simulink model "eVTOL_PX4_2023b"  (R2024b)
settings: Solver=ode4  StartTime=0  StopTime=inf  FixedStep=0.01  RelTol=1e-3
values from neighbouring files (symbols this model uses):
  aDl =     [initdata.mat]
  aDr =     [initdata.mat]
  aDyn =     [initdata.mat]
  Airport = init_airport('PHNL')    [initdata_HIL_eVTOL.m]
  aLat =     [initdata.mat]
  aLon =     [initdata.mat]
  D = Prop.D    [EOM_dt_MC.m]    (also in EOM_get_alf_dt_de_prop_evtol.m = CD * QS)
  dt0 = X(2)    [EOM_get_alf_dt_de_prop_evtol.m]    (also in initdata.mat = 0.258252593971; initdata_HIL_eVTOL.m = EOM_dt_MC)
  EAS0 = TAS0 / EAS2TAS    [initdata_HIL_eVTOL.m]
  FCS = init_FCS    [initdata_HIL_eVTOL.m]
  General = init_layoutdata    [EOM_dt_MC.m]    (also in build_optimized_CA.m; initdata.mat = ; initdata_HIL_eVTOL.m)
  h0 = Con(1)    [EOM_get_alf_dt_de_prop_evtol.m]    (also in initdata.mat = 450; initdata_HIL_eVTOL.m = 50)
  mass = Con(3)    [EOM_get_alf_dt_de_prop_evtol.m]    (also in initdata.mat = 2255.54; initdata_HIL_eVTOL.m = 7)
  Motor = init_motor_evtol    [EOM_dt_MC.m]    (also in initdata.mat = []; initdata_HIL_eVTOL.m)
  Prop = init_propeller_evtol_new    [EOM_dt_MC.m]    (also in initdata_HIL_eVTOL.m)
  R2D = 180/pi    (= 57.2957795131)    [EOM_get_alf_dt_de_prop_evtol.m]    (also in init_FCS.m; init_aerodata_evtol.m; init_airport.m; initdata.mat)
  SAMPLE_TIME = 0.01    [initdata_HIL_eVTOL.m]
  theta0 = -0.0510981441662    [initdata.mat]
undefined symbols (not defined in the file or in its folder): A1, aDa, aDe, aero, asbhl20env, B1, C1, de0, Earth, Environment, INIT_Data, InitData, Kd, Kp, magnitude, Newton, pProp, Raphson, Tc, WGS84
libraries: simulink_extras x63, vrlib x48, sharedtransform x28, simulink x22, slpidlib x20, sharedutil x20, matrix_library x18, aerolibwindfilters x12, aerolibobsolete x8, aerolibasang x8, aerolibatmos2 x6, aerolibfltsims x6
(part 11 of 17)

== system eVTOL_PX4_2023b/FCS/FW/TECS/TECS PX4 & AP201/throttlec_AP201 ==
  LonMod : Inport
  SPE_RATE_C : Inport  Port=2
  SKE_RATE_C : Inport  Port=3
  SPE_RATE : Inport  Port=4
  SKE_RATE : Inport  Port=5
  Add2 : Sum  Inputs=++|
  Add6 : Sum  Inputs=++|
  Add7 : Sum  Inputs=++|
  Add9 : Sum  Inputs=+-|
  Detect Change : simulink/Logic and Bit Operations/Detect Change  vinit=0  OutDataTypeStr=boolean
  Divide2 : Product  Inputs=*/
  Integrator1 : Integrator  ExternalReset=either  LimitOutput=on  UpperSaturationLimit=0.5  LowerSaturationLimit=-0.5  ZeroCross=off
  KTI : Gain  Gain=0.8
  KTP : Gain  Gain=0.4
  PX4 1st order filter (time depended)1 : CustomLib/PX4 1st order filter (time depended)  Commented=on  Ts=0.2
  Rate Limiter Dynamic1 : simulink/Discontinuities/Rate Limiter Dynamic
  Saturation Dynamic : simulink/Discontinuities/Saturation Dynamic  OutMin=[]  OutMax=[]  OutDataTypeStr=Inherit: Same as second input  OutDataType=fixdt(1, 16)  OutScaling=2^-10  DoSatur=off
  Saturation3 : Saturate  UpperLimit=1  LowerLimit=-1
  dE_dot scp : Scope
  dt scp{2..5} (4 alike) : Scope
  dt_slew : Constant  Value=0.8
  dti scp1 : Scope  NumInputPorts=2
  g12 : Gain  Gain=9.8
  g13 : Gain  Gain=-1
  dt : Outport  VectorParamsAs1DForOutWhenUnconnected=off
  wires:
  Add2/1 -> Rate Limiter Dynamic1/2  "dt"
  Saturation Dynamic/1 -> dt scp4/1, Add9/1  "STE_rate_c"
  Rate Limiter Dynamic1/1 -> Saturation3/1
  [STE_rate_min] -> Saturation Dynamic/3
  Add7/1 -> dt scp5/1, Saturation Dynamic/2  "STE_rate_c"
  Divide2/1 -> dE_dot scp/1, KTI/1, KTP/1  "dE_dot"
  g12/1 -> Divide2/2
  SPE_RATE/1 -> Add6/1
  Add9/1 -> Divide2/1  "STE_rate_err"
  [V] -> g12/1
  KTI/1 -> Integrator1/1
  SKE_RATE/1 -> Add6/2
  KTP/1 -> Add2/2, dti scp1/2
  Add6/1 -> dt scp3/1, Add9/2  "STE_rate"
  SKE_RATE_C/1 -> Add7/2
  SPE_RATE_C/1 -> Add7/1
  [STE_rate_max] -> Saturation Dynamic/1
  Integrator1/1 -> Add2/1, dti scp1/1
  dt_slew/1 -> Rate Limiter Dynamic1/1, g13/1
  g13/1 -> Rate Limiter Dynamic1/3
  Saturation3/1 -> dt/1, dt scp2/1
  LonMod/1 -> Detect Change/1
  Detect Change/1 -> Integrator1/2

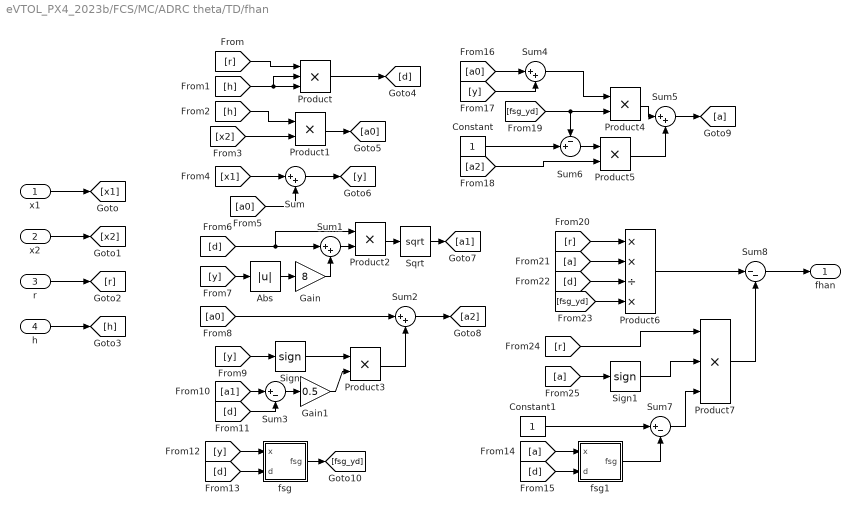
== system eVTOL_PX4_2023b/FCS/MC/ADRC theta/TD/fhan ==
  x1 : Inport
  x2 : Inport  Port=2
  r : Inport  Port=3
  h : Inport  Port=4
  Abs : Abs  SaturateOnIntegerOverflow=off
  Constant : Constant
  Constant1 : Constant
  Gain : Gain  Gain=8
  Gain1 : Gain  Gain=0.5
  Product : Product  Inputs=3
  Product{1..5} (5 alike) : Product
  Product6 : Product  Inputs=**/*
  Product7 : Product  Inputs=***
  Sign : Signum
  Sign1 : Signum
  Sqrt : Sqrt
  Sum{,1..2,4..5} (5 alike) : Sum  Inputs=|++
  Sum3 : Sum  Inputs=|+-
  Sum6 : Sum  Inputs=-+|
  Sum7 : Sum  Inputs=|+-
  Sum8 : Sum  Inputs=|--
  fsg : Subsystem
  fsg1 : Subsystem
  fhan : Outport
  wires:
  Product/1 -> [d]
  x1/1 -> [x1]
  x2/1 -> [x2]
  r/1 -> [r]
  h/1 -> [h]
  [r] -> Product/1
  [h] -> Product/3, Product/2
  [h] -> Product1/1
  [x2] -> Product1/2
  Product1/1 -> [a0]
  [x1] -> Sum/1
  [a0] -> Sum/2
  Sum/1 -> [y]
  [d] -> Sum1/1, Product2/1
  [y] -> Abs/1
  Abs/1 -> Gain/1
  Gain/1 -> Sum1/2
  Sum1/1 -> Product2/2
  Product2/1 -> Sqrt/1
  [a0] -> Sum2/1
  [y] -> Sign/1
  Sign/1 -> Product3/1
  [a1] -> Sum3/1
  [d] -> Sum3/2
  Sum3/1 -> Gain1/1
  Gain1/1 -> Product3/2
  Product3/1 -> Sum2/2
  Sum2/1 -> [a2]
  [y] -> fsg/1(x)
  [d] -> fsg/2(d)
  [d] -> fsg1/2(d)
  [a] -> fsg1/1(x)
  [a0] -> Sum4/1
  [y] -> Sum4/2
  Sum4/1 -> Product4/1
  Product4/1 -> Sum5/1
  [a2] -> Product5/2
  Constant/1 -> Sum6/2
  Sum6/1 -> Product5/1
  Product5/1 -> Sum5/2
  Sum5/1 -> [a]
  fsg/1(fsg) -> [fsg_yd]
  [fsg_yd] -> Sum6/1, Product4/2
  [r] -> Product6/1
  [a] -> Product6/2
  [d] -> Product6/3
  [fsg_yd] -> Product6/4
  Constant1/1 -> Sum7/1
  fsg1/1(fsg) -> Sum7/2
  [a] -> Sign1/1
  [r] -> Product7/1
  Sign1/1 -> Product7/2
  Sum7/1 -> Product7/3
  Product6/1 -> Sum8/1
  Product7/1 -> Sum8/2
  Sum8/1 -> fhan/1
  Sqrt/1 -> [a1]

== system eVTOL_PX4_2023b/Subsystem1/Energy & Power/thrust_1/Propeller /Subsystem ==
  V : Inport
  rpm : Inport  Port=2
  Diameter : Constant  Value=Prop.D
  Divide : Product  Inputs=*//
  Gain : Gain  Gain=1/60
  J : Outport  VectorParamsAs1DForOutWhenUnconnected=off
  wires:
  Divide/1 -> J/1
  V/1 -> Divide/1
  rpm/1 -> Gain/1
  Gain/1 -> Divide/3  "rps"
  Diameter/1 -> Divide/2

== system eVTOL_PX4_2023b/Subsystem1/Energy & Power/thrust_2/Propeller /Subsystem ==
  V : Inport
  rpm : Inport  Port=2
  Diameter : Constant  Value=Prop.D
  Divide : Product  Inputs=*//
  Gain : Gain  Gain=1/60
  J : Outport  VectorParamsAs1DForOutWhenUnconnected=off
  wires:
  Divide/1 -> J/1
  V/1 -> Divide/1
  rpm/1 -> Gain/1
  Gain/1 -> Divide/3  "rps"
  Diameter/1 -> Divide/2

== system eVTOL_PX4_2023b/Subsystem1/Energy & Power/thrust_3/Propeller /Subsystem ==
  V : Inport
  rpm : Inport  Port=2
  Diameter : Constant  Value=Prop.D
  Divide : Product  Inputs=*//
  Gain : Gain  Gain=1/60
  J : Outport  VectorParamsAs1DForOutWhenUnconnected=off
  wires:
  Divide/1 -> J/1
  V/1 -> Divide/1
  rpm/1 -> Gain/1
  Gain/1 -> Divide/3  "rps"
  Diameter/1 -> Divide/2

== system eVTOL_PX4_2023b/Subsystem1/Energy & Power/thrust_4/Propeller /Subsystem ==
  V : Inport
  rpm : Inport  Port=2
  Diameter : Constant  Value=Prop.D
  Divide : Product  Inputs=*//
  Gain : Gain  Gain=1/60
  J : Outport  VectorParamsAs1DForOutWhenUnconnected=off
  wires:
  Divide/1 -> J/1
  V/1 -> Divide/1
  rpm/1 -> Gain/1
  Gain/1 -> Divide/3  "rps"
  Diameter/1 -> Divide/2

== system eVTOL_PX4_2023b/Subsystem1/Energy & Power/thrust_5/Propeller /Subsystem ==
  V : Inport
  rpm : Inport  Port=2
  Diameter : Constant  Value=Prop.D
  Divide : Product  Inputs=*//
  Gain : Gain  Gain=1/60
  J : Outport  VectorParamsAs1DForOutWhenUnconnected=off
  wires:
  Divide/1 -> J/1
  V/1 -> Divide/1
  rpm/1 -> Gain/1
  Gain/1 -> Divide/3  "rps"
  Diameter/1 -> Divide/2

== system eVTOL_PX4_2023b/Subsystem1/Energy & Power/thrust_6/Propeller /Subsystem ==
  V : Inport
  rpm : Inport  Port=2
  Diameter : Constant  Value=Prop.D
  Divide : Product  Inputs=*//
  Gain : Gain  Gain=1/60
  J : Outport  VectorParamsAs1DForOutWhenUnconnected=off
  wires:
  Divide/1 -> J/1
  V/1 -> Divide/1
  rpm/1 -> Gain/1
  Gain/1 -> Divide/3  "rps"
  Diameter/1 -> Divide/2

== system eVTOL_PX4_2023b/Subsystem1/Energy & Power1/thrust_1/Propeller /Subsystem ==
  V : Inport
  rpm : Inport  Port=2
  Diameter : Constant  Value=Prop.D
  Divide : Product  Inputs=*//
  Gain : Gain  Gain=1/60
  J : Outport  VectorParamsAs1DForOutWhenUnconnected=off
  wires:
  Divide/1 -> J/1
  V/1 -> Divide/1
  rpm/1 -> Gain/1
  Gain/1 -> Divide/3  "rps"
  Diameter/1 -> Divide/2

== system eVTOL_PX4_2023b/Subsystem1/Energy & Power1/thrust_2/Propeller /Subsystem ==
  V : Inport
  rpm : Inport  Port=2
  Diameter : Constant  Value=Prop.D
  Divide : Product  Inputs=*//
  Gain : Gain  Gain=1/60
  J : Outport  VectorParamsAs1DForOutWhenUnconnected=off
  wires:
  Divide/1 -> J/1
  V/1 -> Divide/1
  rpm/1 -> Gain/1
  Gain/1 -> Divide/3  "rps"
  Diameter/1 -> Divide/2

== system eVTOL_PX4_2023b/Subsystem1/Energy & Power1/thrust_3/Propeller /Subsystem ==
  V : Inport
  rpm : Inport  Port=2
  Diameter : Constant  Value=Prop.D
  Divide : Product  Inputs=*//
  Gain : Gain  Gain=1/60
  J : Outport  VectorParamsAs1DForOutWhenUnconnected=off
  wires:
  Divide/1 -> J/1
  V/1 -> Divide/1
  rpm/1 -> Gain/1
  Gain/1 -> Divide/3  "rps"
  Diameter/1 -> Divide/2

== system eVTOL_PX4_2023b/Subsystem1/Energy & Power1/thrust_4/Propeller /Subsystem ==
  V : Inport
  rpm : Inport  Port=2
  Diameter : Constant  Value=Prop.D
  Divide : Product  Inputs=*//
  Gain : Gain  Gain=1/60
  J : Outport  VectorParamsAs1DForOutWhenUnconnected=off
  wires:
  Divide/1 -> J/1
  V/1 -> Divide/1
  rpm/1 -> Gain/1
  Gain/1 -> Divide/3  "rps"
  Diameter/1 -> Divide/2

== system eVTOL_PX4_2023b/Subsystem1/Energy & Power1/thrust_5/Propeller /Subsystem ==
  V : Inport
  rpm : Inport  Port=2
  Diameter : Constant  Value=Prop.D
  Divide : Product  Inputs=*//
  Gain : Gain  Gain=1/60
  J : Outport  VectorParamsAs1DForOutWhenUnconnected=off
  wires:
  Divide/1 -> J/1
  V/1 -> Divide/1
  rpm/1 -> Gain/1
  Gain/1 -> Divide/3  "rps"
  Diameter/1 -> Divide/2

== system eVTOL_PX4_2023b/Subsystem1/Energy & Power1/thrust_6/Propeller /Subsystem ==
  V : Inport
  rpm : Inport  Port=2
  Diameter : Constant  Value=Prop.D
  Divide : Product  Inputs=*//
  Gain : Gain  Gain=1/60
  J : Outport  VectorParamsAs1DForOutWhenUnconnected=off
  wires:
  Divide/1 -> J/1
  V/1 -> Divide/1
  rpm/1 -> Gain/1
  Gain/1 -> Divide/3  "rps"
  Diameter/1 -> Divide/2

== system eVTOL_PX4_2023b/Subsystem1/Environment/Wind Models/Dryden Wind Turbulence Model (Continuous (+q -r))/Angle Conversion ==
  in : Inport  Unit=deg
  Unit Conversion : UnitConversion
  out : Outport  Unit=rad  VectorParamsAs1DForOutWhenUnconnected=off
  wires:
  in/1 -> Unit Conversion/1
  Unit Conversion/1 -> out/1

== system eVTOL_PX4_2023b/Subsystem1/Environment/Wind Models/Dryden Wind Turbulence Model (Continuous (+q -r))/Filters on angular rates ==
  vg : Inport
  wg : Inport  Port=2
  V : Inport  Port=3  Unit=ft/s
  Lw : Inport  Port=4
  sigma_w : Inport  Port=5
  Noise : Inport  Port=6
  wingspan : Inport  Port=7
  Constant1 : Constant  Value=T_on
  Constant2 : Constant  Value=T_on
  Constant3 : Constant  Value=T_on
  Hpgw : aerolibwindfilters/Hpgw(s)  SystemSampleTime=-1  VariantActivationTime=update diagram  AllowFlexibleInterface=on  Latency=0  AutoFrameSizeCalculation=off
  Hqgw : aerolibwindfilters/Hqgw(s) (+q)  SystemSampleTime=-1  VariantActivationTime=update diagram  AllowFlexibleInterface=on  Latency=0  AutoFrameSizeCalculation=off
  Hrgw : aerolibwindfilters/Hrgw(s) (-r)  SystemSampleTime=-1  VariantActivationTime=update diagram  AllowFlexibleInterface=on  Latency=0  AutoFrameSizeCalculation=off
  pgw : Outport  InitialOutput=0  VectorParamsAs1DForOutWhenUnconnected=off
  qgw : Outport  Port=2  InitialOutput=0  VectorParamsAs1DForOutWhenUnconnected=off
  rgw : Outport  Port=3  InitialOutput=0  VectorParamsAs1DForOutWhenUnconnected=off
  wires:
  Constant3/1 -> Hrgw/Enable
  Constant2/1 -> Hqgw/Enable
  Constant1/1 -> Hpgw/Enable
  Noise/1 -> Hpgw/3
  Lw/1 -> Hpgw/1
  sigma_w/1 -> Hpgw/2
  V/1 -> Hpgw/4, Hqgw/1, Hrgw/1
  Hpgw/1 -> pgw/1
  wg/1 -> Hqgw/2
  Hqgw/1 -> qgw/1
  Hrgw/1 -> rgw/1
  vg/1 -> Hrgw/2
  wingspan/1 -> Hqgw/3, Hrgw/3, Hpgw/5

== system eVTOL_PX4_2023b/Subsystem1/Environment/Wind Models/Dryden Wind Turbulence Model (Continuous (+q -r))/Length Conversion ==
  in : Inport
  Unit Conversion : UnitConversion
  out : Outport  Unit=ft  VectorParamsAs1DForOutWhenUnconnected=off
  wires:
  in/1 -> Unit Conversion/1
  Unit Conversion/1 -> out/1

== system eVTOL_PX4_2023b/Subsystem1/Environment/Wind Models/Dryden Wind Turbulence Model (Continuous (+q -r))/Length Conversion1 ==
  in : Inport  Unit=m
  Unit Conversion : UnitConversion
  out : Outport  Unit=ft  VectorParamsAs1DForOutWhenUnconnected=off
  wires:
  in/1 -> Unit Conversion/1
  Unit Conversion/1 -> out/1

== system eVTOL_PX4_2023b/Subsystem1/Environment/Wind Models/Dryden Wind Turbulence Model (Continuous (+q -r))/RMS turbulence intensities ==
  Altitude : Inport
  Windspeed at 20ft (6m) : Inport  Port=2
  High Altitude Intensity : Subsystem
  Low Altitude Intensity : Subsystem
  Mux1 : Mux  Inputs=2
  Mux2 : Mux  Inputs=2
  "sigma_ug " : Outport  VectorParamsAs1DForOutWhenUnconnected=off
  sigma_vg : Outport  Port=2  VectorParamsAs1DForOutWhenUnconnected=off
  sigma_wg : Outport  Port=3  VectorParamsAs1DForOutWhenUnconnected=off
  wires:
  Mux2/1 -> sigma_vg/1, "sigma_ug "/1  "sigmaug"
  Windspeed at 20ft (6m)/1 -> Low Altitude Intensity/1(Windspeed at 20ft (6m))
  High Altitude Intensity/1(sigma_ug sigma_vg sigma_wg) -> Mux2/2, Mux1/2
  Mux1/1 -> sigma_wg/1  "sigmawg"
  Low Altitude Intensity/2(sigma_wg) -> Mux1/1
  Low Altitude Intensity/1(sigma_ug sigma_vg) -> Mux2/1
  Altitude/1 -> High Altitude Intensity/1(h), Low Altitude Intensity/2(h)

== system eVTOL_PX4_2023b/Subsystem1/Environment/Wind Models/Dryden Wind Turbulence Model (Continuous (+q -r))/Select angular rates ==
  pgw_h&l : Inport
  qgw_h&l : Inport  Port=2
  rgw_h&l : Inport  Port=3
  "DCM, altitude, Wdeg" : Inport  Port=4
  Bus Creator : BusCreator  Inputs=6
  Bus Selector : BusSelector  OutputSignals=pgw,qgw,rgw
  Bus Selector1 : BusSelector  OutputSignals=pgw,qgw,rgw,DCM,Wdeg,altitude
  Bus Selector2 : BusSelector  OutputSignals=DCM,pgw,qgw,rgw,Wdeg
  Bus Selector3 : BusSelector  OutputSignals=altitude,DCM,Wdeg
  Interpolate rates : Subsystem  TreatAsAtomicUnit=on
  Low altitude rates : Subsystem  TreatAsAtomicUnit=on
  Medium/High altitude rates : Subsystem  TreatAsAtomicUnit=on
  Merge Subsystems : Subsystem
  "if Height < Max low altitude elseif Height > Min isotropic altitude " : If  IfExpression=u1<=max_height_low  ElseIfExpressions=u1>=min_height_high
  pgw : Outport  InitialOutput=0  VectorParamsAs1DForOutWhenUnconnected=off
  qgw : Outport  Port=2  InitialOutput=0  VectorParamsAs1DForOutWhenUnconnected=off
  rgw : Outport  Port=3  InitialOutput=0  VectorParamsAs1DForOutWhenUnconnected=off
  wires:
  "DCM, altitude, Wdeg"/1 -> Bus Selector3/1
  Bus Selector3/1 -> Bus Creator/1, "if Height < Max low altitude elseif Height > Min isotropic altitude "/1  "<altitude>"
  Bus Creator/1 -> Bus Selector2/1, Bus Selector1/1, Bus Selector/1
  Bus Selector3/2 -> Bus Creator/2  "<DCM>"
  pgw_h&l/1 -> Bus Creator/3
  qgw_h&l/1 -> Bus Creator/4
  rgw_h&l/1 -> Bus Creator/5
  Bus Selector1/1 -> Interpolate rates/1(pgw_h&l)  "<pgw>"
  Bus Selector1/2 -> Interpolate rates/2(qgw_h&l)  "<qgw>"
  Bus Selector1/3 -> Interpolate rates/3(rgw_h&l)  "<rgw>"
  Bus Selector1/4 -> Interpolate rates/4(DCM)  "<DCM>"
  Bus Selector1/6 -> Interpolate rates/6(Altitude)  "<altitude>"
  Bus Selector2/1 -> Low altitude rates/1(DCM)  "<DCM>"
  Bus Selector2/2 -> Low altitude rates/2(pgw_h&l)  "<pgw>"
  Bus Selector2/3 -> Low altitude rates/3(qgw_h&l)  "<qgw>"
  Bus Selector2/4 -> Low altitude rates/4(rgw_h&l)  "<rgw>"
  Bus Selector/1 -> Medium/High altitude rates/1(pgw_h&l)  "<pgw>"
  Bus Selector/2 -> Medium/High altitude rates/2(qgw_h&l)  "<qgw>"
  Bus Selector/3 -> Medium/High altitude rates/3(rgw_h&l)  "<rgw>"
  Merge Subsystems/1(pgw) -> pgw/1
  Merge Subsystems/2(qgw) -> qgw/1
  Merge Subsystems/3(rgw) -> rgw/1
  Interpolate rates/1(pgw,qgw,rgw) -> Merge Subsystems/3(interpolated)
  Bus Selector3/3 -> Bus Creator/6  "<Wdeg>"
  Bus Selector2/5 -> Low altitude rates/5(Wind direction)  "<Wdeg>"
  Bus Selector1/5 -> Interpolate rates/5(Wind direction)  "<Wdeg>"
  "if Height < Max low altitude elseif Height > Min isotropic altitude "/1 -> [IF]
  [IF] -> Low altitude rates/Action
  "if Height < Max low altitude elseif Height > Min isotropic altitude "/2 -> [ELSEIF]
  [ELSEIF] -> Medium/High altitude rates/Action
  [ELSE] -> Interpolate rates/Action
  "if Height < Max low altitude elseif Height > Min isotropic altitude "/3 -> [ELSE]
  Medium/High altitude rates/1(pgw,qgw,rgw) -> Merge Subsystems/2(high)
  Low altitude rates/1(pgw,qgw,rgw) -> Merge Subsystems/1(low)

== system eVTOL_PX4_2023b/Subsystem1/Environment/Wind Models/Dryden Wind Turbulence Model (Continuous (+q -r))/Select velocities ==
  "DCM, altitude, Wdeg" : Inport
  ugw_h&l : Inport  Port=2
  vgw_h&l : Inport  Port=3
  wgw_h&l : Inport  Port=4
  Bus Creator : BusCreator  Inputs=6
  Bus Selector : BusSelector  OutputSignals=ugw,vgw,wgw
  Bus Selector1 : BusSelector  OutputSignals=ugw,vgw,wgw,DCM,Wdeg,altitude
  Bus Selector2 : BusSelector  OutputSignals=DCM,ugw,vgw,wgw,Wdeg
  Bus Selector3 : BusSelector  OutputSignals=altitude,DCM,Wdeg
  Interpolate velocities : Subsystem  TreatAsAtomicUnit=on
  Low altitude velocities : Subsystem  TreatAsAtomicUnit=on
  Medium/High altitude velocities : Subsystem  TreatAsAtomicUnit=on
  Merge Subsystems : Subsystem
  "if Height < Max low altitude elseif Height > Min isotropic altitude " : If  IfExpression=u1<=max_height_low  ElseIfExpressions=u1>=min_height_high
  ugw : Outport  Unit=ft/s  InitialOutput=0  VectorParamsAs1DForOutWhenUnconnected=off
  vgw : Outport  Port=2  Unit=ft/s  InitialOutput=0  VectorParamsAs1DForOutWhenUnconnected=off
  wgw : Outport  Port=3  Unit=ft/s  InitialOutput=0  VectorParamsAs1DForOutWhenUnconnected=off
  wires:
  "DCM, altitude, Wdeg"/1 -> Bus Selector3/1
  Bus Selector1/6 -> Interpolate velocities/6(Altitude)  "<altitude>"
  Low altitude velocities/1(ugw,vgw,wgw) -> Merge Subsystems/1(low)
  Medium/High altitude velocities/1(ugw,vgw,wgw) -> Merge Subsystems/2(high)
  "if Height < Max low altitude elseif Height > Min isotropic altitude "/3 -> [ELSE]
  [ELSE] -> Interpolate velocities/Action
  [ELSEIF] -> Medium/High altitude velocities/Action
  "if Height < Max low altitude elseif Height > Min isotropic altitude "/2 -> [ELSEIF]
  [IF] -> Low altitude velocities/Action
  "if Height < Max low altitude elseif Height > Min isotropic altitude "/1 -> [IF]
  Bus Selector1/5 -> Interpolate velocities/5(Wind direction)  "<Wdeg>"
  Bus Selector2/5 -> Low altitude velocities/5(Wind direction)  "<Wdeg>"
  Bus Selector3/3 -> Bus Creator/6  "<Wdeg>"
  Interpolate velocities/1(ugw,vgw,wgw) -> Merge Subsystems/3(interpolated)
  Merge Subsystems/3(wgw) -> wgw/1
  Merge Subsystems/2(vgw) -> vgw/1
  Merge Subsystems/1(ugw) -> ugw/1
  Bus Selector/3 -> Medium/High altitude velocities/3(wgw_h&l)  "<wgw>"
  Bus Selector/2 -> Medium/High altitude velocities/2(vgw_h&l)  "<vgw>"
  Bus Selector/1 -> Medium/High altitude velocities/1(ugw_h&l)  "<ugw>"
  Bus Selector2/4 -> Low altitude velocities/4(wgw_h&l)  "<wgw>"
  Bus Selector2/3 -> Low altitude velocities/3(vgw_h&l)  "<vgw>"
  Bus Selector2/2 -> Low altitude velocities/2(ugw_h&l)  "<ugw>"
  Bus Selector2/1 -> Low altitude velocities/1(DCM)  "<DCM>"
  Bus Selector1/4 -> Interpolate velocities/4(DCM)  "<DCM>"
  Bus Selector1/3 -> Interpolate velocities/3(wgw_h&l)  "<wgw>"
  Bus Selector1/2 -> Interpolate velocities/2(vgw_h&l)  "<vgw>"
  Bus Selector1/1 -> Interpolate velocities/1(ugw_h&l)  "<ugw>"
  wgw_h&l/1 -> Bus Creator/5
  vgw_h&l/1 -> Bus Creator/4
  ugw_h&l/1 -> Bus Creator/3
  Bus Selector3/2 -> Bus Creator/2  "<DCM>"
  Bus Creator/1 -> Bus Selector2/1, Bus Selector/1, Bus Selector1/1
  Bus Selector3/1 -> Bus Creator/1, "if Height < Max low altitude elseif Height > Min isotropic altitude "/1  "<altitude>"

== system eVTOL_PX4_2023b/Subsystem1/Environment/Wind Models/Dryden Wind Turbulence Model (Continuous (+q -r))/Turbulence scale lengths ==
  Altitude : Inport
  Low altitude scale length : Subsystem
  Lv : Gain  SaturateOnIntegerOverflow=on  OutDataTypeStr=Inherit: Same as input  ParamDataTypeStr=Inherit: Same as input
  Lw : Gain  SaturateOnIntegerOverflow=on  OutDataTypeStr=Inherit: Same as input  ParamDataTypeStr=Inherit: Same as input
  Medium/High altitude scale length : Subsystem
  Mux : Mux  Inputs=2
  Mux1 : Mux  Inputs=2
  L_ug : Outport  VectorParamsAs1DForOutWhenUnconnected=off
  L_vg : Outport  Port=2  VectorParamsAs1DForOutWhenUnconnected=off
  L_wg : Outport  Port=3  VectorParamsAs1DForOutWhenUnconnected=off
  wires:
  Lv/1 -> L_vg/1
  Lw/1 -> L_wg/1
  Altitude/1 -> Low altitude scale length/1(h)
  Mux/1 -> Lw/1  "Lwg"
  Mux1/1 -> Lv/1, L_ug/1  "Lug"
  Low altitude scale length/1(L_ug L_vg) -> Mux1/1
  Low altitude scale length/2(L_wg) -> Mux/1
  Medium/High altitude scale length/1(L_ug L_vg L_wg) -> Mux1/2, Mux/2

== system eVTOL_PX4_2023b/Subsystem1/Environment/Wind Models/Dryden Wind Turbulence Model (Continuous (+q -r))/Velocity Conversion ==
  in : Inport
  Unit Conversion : UnitConversion
  out : Outport  Unit=ft/s  VectorParamsAs1DForOutWhenUnconnected=off
  wires:
  in/1 -> Unit Conversion/1
  Unit Conversion/1 -> out/1

== system eVTOL_PX4_2023b/Subsystem1/Environment/Wind Models/Dryden Wind Turbulence Model (Continuous (+q -r))/Velocity Conversion2 ==
  in : Inport  Unit=m/s
  Unit Conversion : UnitConversion
  out : Outport  Unit=ft/s  VectorParamsAs1DForOutWhenUnconnected=off
  wires:
  in/1 -> Unit Conversion/1
  Unit Conversion/1 -> out/1

== system eVTOL_PX4_2023b/Subsystem1/Environment1/Wind Models/Dryden Wind Turbulence Model (Continuous (+q -r))/Angle Conversion ==
  in : Inport  Unit=deg
  Unit Conversion : UnitConversion
  out : Outport  Unit=rad  VectorParamsAs1DForOutWhenUnconnected=off
  wires:
  in/1 -> Unit Conversion/1
  Unit Conversion/1 -> out/1

== system eVTOL_PX4_2023b/Subsystem1/Environment1/Wind Models/Dryden Wind Turbulence Model (Continuous (+q -r))/Filters on angular rates ==
  vg : Inport
  wg : Inport  Port=2
  V : Inport  Port=3  Unit=ft/s
  Lw : Inport  Port=4
  sigma_w : Inport  Port=5
  Noise : Inport  Port=6
  wingspan : Inport  Port=7
  Constant1 : Constant  Value=T_on
  Constant2 : Constant  Value=T_on
  Constant3 : Constant  Value=T_on
  Hpgw : aerolibwindfilters/Hpgw(s)  SystemSampleTime=-1  VariantActivationTime=update diagram  AllowFlexibleInterface=on  Latency=0  AutoFrameSizeCalculation=off
  Hqgw : aerolibwindfilters/Hqgw(s) (+q)  SystemSampleTime=-1  VariantActivationTime=update diagram  AllowFlexibleInterface=on  Latency=0  AutoFrameSizeCalculation=off
  Hrgw : aerolibwindfilters/Hrgw(s) (-r)  SystemSampleTime=-1  VariantActivationTime=update diagram  AllowFlexibleInterface=on  Latency=0  AutoFrameSizeCalculation=off
  pgw : Outport  InitialOutput=0  VectorParamsAs1DForOutWhenUnconnected=off
  qgw : Outport  Port=2  InitialOutput=0  VectorParamsAs1DForOutWhenUnconnected=off
  rgw : Outport  Port=3  InitialOutput=0  VectorParamsAs1DForOutWhenUnconnected=off
  wires:
  Constant3/1 -> Hrgw/Enable
  Constant2/1 -> Hqgw/Enable
  Constant1/1 -> Hpgw/Enable
  Noise/1 -> Hpgw/3
  Lw/1 -> Hpgw/1
  sigma_w/1 -> Hpgw/2
  V/1 -> Hpgw/4, Hqgw/1, Hrgw/1
  Hpgw/1 -> pgw/1
  wg/1 -> Hqgw/2
  Hqgw/1 -> qgw/1
  Hrgw/1 -> rgw/1
  vg/1 -> Hrgw/2
  wingspan/1 -> Hqgw/3, Hrgw/3, Hpgw/5

== system eVTOL_PX4_2023b/Subsystem1/Environment1/Wind Models/Dryden Wind Turbulence Model (Continuous (+q -r))/Length Conversion ==
  in : Inport
  Unit Conversion : UnitConversion
  out : Outport  Unit=ft  VectorParamsAs1DForOutWhenUnconnected=off
  wires:
  in/1 -> Unit Conversion/1
  Unit Conversion/1 -> out/1

== system eVTOL_PX4_2023b/Subsystem1/Environment1/Wind Models/Dryden Wind Turbulence Model (Continuous (+q -r))/Length Conversion1 ==
  in : Inport  Unit=m
  Unit Conversion : UnitConversion
  out : Outport  Unit=ft  VectorParamsAs1DForOutWhenUnconnected=off
  wires:
  in/1 -> Unit Conversion/1
  Unit Conversion/1 -> out/1

== system eVTOL_PX4_2023b/Subsystem1/Environment1/Wind Models/Dryden Wind Turbulence Model (Continuous (+q -r))/RMS turbulence intensities ==
  Altitude : Inport
  Windspeed at 20ft (6m) : Inport  Port=2
  High Altitude Intensity : Subsystem
  Low Altitude Intensity : Subsystem
  Mux1 : Mux  Inputs=2
  Mux2 : Mux  Inputs=2
  "sigma_ug " : Outport  VectorParamsAs1DForOutWhenUnconnected=off
  sigma_vg : Outport  Port=2  VectorParamsAs1DForOutWhenUnconnected=off
  sigma_wg : Outport  Port=3  VectorParamsAs1DForOutWhenUnconnected=off
  wires:
  Mux2/1 -> sigma_vg/1, "sigma_ug "/1  "sigmaug"
  Windspeed at 20ft (6m)/1 -> Low Altitude Intensity/1(Windspeed at 20ft (6m))
  High Altitude Intensity/1(sigma_ug sigma_vg sigma_wg) -> Mux2/2, Mux1/2
  Mux1/1 -> sigma_wg/1  "sigmawg"
  Low Altitude Intensity/2(sigma_wg) -> Mux1/1
  Low Altitude Intensity/1(sigma_ug sigma_vg) -> Mux2/1
  Altitude/1 -> High Altitude Intensity/1(h), Low Altitude Intensity/2(h)

== system eVTOL_PX4_2023b/Subsystem1/Environment1/Wind Models/Dryden Wind Turbulence Model (Continuous (+q -r))/Select angular rates ==
  pgw_h&l : Inport
  qgw_h&l : Inport  Port=2
  rgw_h&l : Inport  Port=3
  "DCM, altitude, Wdeg" : Inport  Port=4
  Bus Creator : BusCreator  Inputs=6
  Bus Selector : BusSelector  OutputSignals=pgw,qgw,rgw
  Bus Selector1 : BusSelector  OutputSignals=pgw,qgw,rgw,DCM,Wdeg,altitude
  Bus Selector2 : BusSelector  OutputSignals=DCM,pgw,qgw,rgw,Wdeg
  Bus Selector3 : BusSelector  OutputSignals=altitude,DCM,Wdeg
  Interpolate rates : Subsystem  TreatAsAtomicUnit=on
  Low altitude rates : Subsystem  TreatAsAtomicUnit=on
  Medium/High altitude rates : Subsystem  TreatAsAtomicUnit=on
  Merge Subsystems : Subsystem
  "if Height < Max low altitude elseif Height > Min isotropic altitude " : If  IfExpression=u1<=max_height_low  ElseIfExpressions=u1>=min_height_high
  pgw : Outport  InitialOutput=0  VectorParamsAs1DForOutWhenUnconnected=off
  qgw : Outport  Port=2  InitialOutput=0  VectorParamsAs1DForOutWhenUnconnected=off
  rgw : Outport  Port=3  InitialOutput=0  VectorParamsAs1DForOutWhenUnconnected=off
  wires:
  "DCM, altitude, Wdeg"/1 -> Bus Selector3/1
  Bus Selector3/1 -> Bus Creator/1, "if Height < Max low altitude elseif Height > Min isotropic altitude "/1  "<altitude>"
  Bus Creator/1 -> Bus Selector2/1, Bus Selector1/1, Bus Selector/1
  Bus Selector3/2 -> Bus Creator/2  "<DCM>"
  pgw_h&l/1 -> Bus Creator/3
  qgw_h&l/1 -> Bus Creator/4
  rgw_h&l/1 -> Bus Creator/5
  Bus Selector1/1 -> Interpolate rates/1(pgw_h&l)  "<pgw>"
  Bus Selector1/2 -> Interpolate rates/2(qgw_h&l)  "<qgw>"
  Bus Selector1/3 -> Interpolate rates/3(rgw_h&l)  "<rgw>"
  Bus Selector1/4 -> Interpolate rates/4(DCM)  "<DCM>"
  Bus Selector1/6 -> Interpolate rates/6(Altitude)  "<altitude>"
  Bus Selector2/1 -> Low altitude rates/1(DCM)  "<DCM>"
  Bus Selector2/2 -> Low altitude rates/2(pgw_h&l)  "<pgw>"
  Bus Selector2/3 -> Low altitude rates/3(qgw_h&l)  "<qgw>"
  Bus Selector2/4 -> Low altitude rates/4(rgw_h&l)  "<rgw>"
  Bus Selector/1 -> Medium/High altitude rates/1(pgw_h&l)  "<pgw>"
  Bus Selector/2 -> Medium/High altitude rates/2(qgw_h&l)  "<qgw>"
  Bus Selector/3 -> Medium/High altitude rates/3(rgw_h&l)  "<rgw>"
  Merge Subsystems/1(pgw) -> pgw/1
  Merge Subsystems/2(qgw) -> qgw/1
  Merge Subsystems/3(rgw) -> rgw/1
  Interpolate rates/1(pgw,qgw,rgw) -> Merge Subsystems/3(interpolated)
  Bus Selector3/3 -> Bus Creator/6  "<Wdeg>"
  Bus Selector2/5 -> Low altitude rates/5(Wind direction)  "<Wdeg>"
  Bus Selector1/5 -> Interpolate rates/5(Wind direction)  "<Wdeg>"
  "if Height < Max low altitude elseif Height > Min isotropic altitude "/1 -> [IF]
  [IF] -> Low altitude rates/Action
  "if Height < Max low altitude elseif Height > Min isotropic altitude "/2 -> [ELSEIF]
  [ELSEIF] -> Medium/High altitude rates/Action
  [ELSE] -> Interpolate rates/Action
  "if Height < Max low altitude elseif Height > Min isotropic altitude "/3 -> [ELSE]
  Medium/High altitude rates/1(pgw,qgw,rgw) -> Merge Subsystems/2(high)
  Low altitude rates/1(pgw,qgw,rgw) -> Merge Subsystems/1(low)

== system eVTOL_PX4_2023b/Subsystem1/Environment1/Wind Models/Dryden Wind Turbulence Model (Continuous (+q -r))/Select velocities ==
  "DCM, altitude, Wdeg" : Inport
  ugw_h&l : Inport  Port=2
  vgw_h&l : Inport  Port=3
  wgw_h&l : Inport  Port=4
  Bus Creator : BusCreator  Inputs=6
  Bus Selector : BusSelector  OutputSignals=ugw,vgw,wgw
  Bus Selector1 : BusSelector  OutputSignals=ugw,vgw,wgw,DCM,Wdeg,altitude
  Bus Selector2 : BusSelector  OutputSignals=DCM,ugw,vgw,wgw,Wdeg
  Bus Selector3 : BusSelector  OutputSignals=altitude,DCM,Wdeg
  Interpolate velocities : Subsystem  TreatAsAtomicUnit=on
  Low altitude velocities : Subsystem  TreatAsAtomicUnit=on
  Medium/High altitude velocities : Subsystem  TreatAsAtomicUnit=on
  Merge Subsystems : Subsystem
  "if Height < Max low altitude elseif Height > Min isotropic altitude " : If  IfExpression=u1<=max_height_low  ElseIfExpressions=u1>=min_height_high
  ugw : Outport  Unit=ft/s  InitialOutput=0  VectorParamsAs1DForOutWhenUnconnected=off
  vgw : Outport  Port=2  Unit=ft/s  InitialOutput=0  VectorParamsAs1DForOutWhenUnconnected=off
  wgw : Outport  Port=3  Unit=ft/s  InitialOutput=0  VectorParamsAs1DForOutWhenUnconnected=off
  wires:
  "DCM, altitude, Wdeg"/1 -> Bus Selector3/1
  Bus Selector1/6 -> Interpolate velocities/6(Altitude)  "<altitude>"
  Low altitude velocities/1(ugw,vgw,wgw) -> Merge Subsystems/1(low)
  Medium/High altitude velocities/1(ugw,vgw,wgw) -> Merge Subsystems/2(high)
  "if Height < Max low altitude elseif Height > Min isotropic altitude "/3 -> [ELSE]
  [ELSE] -> Interpolate velocities/Action
  [ELSEIF] -> Medium/High altitude velocities/Action
  "if Height < Max low altitude elseif Height > Min isotropic altitude "/2 -> [ELSEIF]
  [IF] -> Low altitude velocities/Action
  "if Height < Max low altitude elseif Height > Min isotropic altitude "/1 -> [IF]
  Bus Selector1/5 -> Interpolate velocities/5(Wind direction)  "<Wdeg>"
  Bus Selector2/5 -> Low altitude velocities/5(Wind direction)  "<Wdeg>"
  Bus Selector3/3 -> Bus Creator/6  "<Wdeg>"
  Interpolate velocities/1(ugw,vgw,wgw) -> Merge Subsystems/3(interpolated)
  Merge Subsystems/3(wgw) -> wgw/1
  Merge Subsystems/2(vgw) -> vgw/1
  Merge Subsystems/1(ugw) -> ugw/1
  Bus Selector/3 -> Medium/High altitude velocities/3(wgw_h&l)  "<wgw>"
  Bus Selector/2 -> Medium/High altitude velocities/2(vgw_h&l)  "<vgw>"
  Bus Selector/1 -> Medium/High altitude velocities/1(ugw_h&l)  "<ugw>"
  Bus Selector2/4 -> Low altitude velocities/4(wgw_h&l)  "<wgw>"
  Bus Selector2/3 -> Low altitude velocities/3(vgw_h&l)  "<vgw>"
  Bus Selector2/2 -> Low altitude velocities/2(ugw_h&l)  "<ugw>"
  Bus Selector2/1 -> Low altitude velocities/1(DCM)  "<DCM>"
  Bus Selector1/4 -> Interpolate velocities/4(DCM)  "<DCM>"
  Bus Selector1/3 -> Interpolate velocities/3(wgw_h&l)  "<wgw>"
  Bus Selector1/2 -> Interpolate velocities/2(vgw_h&l)  "<vgw>"
  Bus Selector1/1 -> Interpolate velocities/1(ugw_h&l)  "<ugw>"
  wgw_h&l/1 -> Bus Creator/5
  vgw_h&l/1 -> Bus Creator/4
  ugw_h&l/1 -> Bus Creator/3
  Bus Selector3/2 -> Bus Creator/2  "<DCM>"
  Bus Creator/1 -> Bus Selector2/1, Bus Selector/1, Bus Selector1/1
  Bus Selector3/1 -> Bus Creator/1, "if Height < Max low altitude elseif Height > Min isotropic altitude "/1  "<altitude>"

== system eVTOL_PX4_2023b/Subsystem1/Environment1/Wind Models/Dryden Wind Turbulence Model (Continuous (+q -r))/Turbulence scale lengths ==
  Altitude : Inport
  Low altitude scale length : Subsystem
  Lv : Gain  SaturateOnIntegerOverflow=on  OutDataTypeStr=Inherit: Same as input  ParamDataTypeStr=Inherit: Same as input
  Lw : Gain  SaturateOnIntegerOverflow=on  OutDataTypeStr=Inherit: Same as input  ParamDataTypeStr=Inherit: Same as input
  Medium/High altitude scale length : Subsystem
  Mux : Mux  Inputs=2
  Mux1 : Mux  Inputs=2
  L_ug : Outport  VectorParamsAs1DForOutWhenUnconnected=off
  L_vg : Outport  Port=2  VectorParamsAs1DForOutWhenUnconnected=off
  L_wg : Outport  Port=3  VectorParamsAs1DForOutWhenUnconnected=off
  wires:
  Lv/1 -> L_vg/1
  Lw/1 -> L_wg/1
  Altitude/1 -> Low altitude scale length/1(h)
  Mux/1 -> Lw/1  "Lwg"
  Mux1/1 -> Lv/1, L_ug/1  "Lug"
  Low altitude scale length/1(L_ug L_vg) -> Mux1/1
  Low altitude scale length/2(L_wg) -> Mux/1
  Medium/High altitude scale length/1(L_ug L_vg L_wg) -> Mux1/2, Mux/2

== system eVTOL_PX4_2023b/Subsystem1/Environment1/Wind Models/Dryden Wind Turbulence Model (Continuous (+q -r))/Velocity Conversion ==
  in : Inport
  Unit Conversion : UnitConversion
  out : Outport  Unit=ft/s  VectorParamsAs1DForOutWhenUnconnected=off
  wires:
  in/1 -> Unit Conversion/1
  Unit Conversion/1 -> out/1

== system eVTOL_PX4_2023b/Subsystem1/Environment1/Wind Models/Dryden Wind Turbulence Model (Continuous (+q -r))/Velocity Conversion2 ==
  in : Inport  Unit=m/s
  Unit Conversion : UnitConversion
  out : Outport  Unit=ft/s  VectorParamsAs1DForOutWhenUnconnected=off
  wires:
  in/1 -> Unit Conversion/1
  Unit Conversion/1 -> out/1

== system eVTOL_PX4_2023b/Subsystem1/airframe/Flight Conditions/Incidence, Sideslip, & Airspeed/Subsystem ==
  V : Inport
  Demux1 : Demux  Outputs=3
      settings: DisplayOption=none
  Terminator : Terminator
  w : Outport  VectorParamsAs1DForOutWhenUnconnected=off
  U : Outport  Port=2  VectorParamsAs1DForOutWhenUnconnected=off
  wires:
  Demux1/3 -> w/1
  Demux1/2 -> Terminator/1
  V/1 -> Demux1/1
  Demux1/1 -> U/1

== system eVTOL_PX4_2023b/Subsystem1/airframe/Flight Conditions/Incidence, Sideslip, & Airspeed/Subsystem1 ==
  V : Inport
  Demux1 : Demux  Outputs=3
      settings: DisplayOption=none
  Terminator : Terminator
  Terminator1 : Terminator
  v : Outport  VectorParamsAs1DForOutWhenUnconnected=off
  wires:
  Demux1/1 -> Terminator/1
  V/1 -> Demux1/1
  Demux1/2 -> v/1
  Demux1/3 -> Terminator1/1

== system eVTOL_PX4_2023b/Subsystem1/airframe/Flight Conditions/Incidence, Sideslip, & Airspeed/dot ==
  Vb : Inport
  Demux1 : Demux  Outputs=3
  Product : Product  RndMeth=Zero
  Product1 : Product  RndMeth=Zero
  Product2 : Product  RndMeth=Zero
  Sum : Sum  Inputs=+++
  dot : Outport  VectorParamsAs1DForOutWhenUnconnected=off
  wires:
  Product2/1 -> Sum/3
  Demux1/3 -> Product2/2, Product2/1
  Product/1 -> Sum/1
  Product1/1 -> Sum/2
  Sum/1 -> dot/1
  Vb/1 -> Demux1/1
  Demux1/1 -> Product/2, Product/1
  Demux1/2 -> Product1/1, Product1/2

== system eVTOL_PX4_2023b/Subsystem1/airframe/force moment/Gear&FM in body axis/F&M  Front Gear Left ==
  PlantData : Inport
  dg : Inport  Port=2
  Bus Selector : BusSelector  OutputSignals=Xe,DCM_be,Vb,pqr,Euler
  Constant1 : Constant  Value=General.CD0_gear_taxi
  Constant{3,5..6,9,11} (5 alike) : Constant  Value=0
  Constant15 : Constant  Value=InitData.h_runway
  Constant2 : Constant  Value=General.pos_fgl
  Constant4 : Constant  Value=General.Kb
  Constant7 : Constant  Value=General.Kf
  Constant8 : Constant  Value=General.Cf
  Cross Product : vrlib/Utilities/Cross Product
  Cross Product1 : vrlib/Utilities/Cross Product
  Divide : Product  Inputs=*/
  F_fgl scp : Scope
  F_in_earth scp : Scope
  F_in_earth scp1 : Scope
  F_in_gear scp : Scope
  Gain1 : Gain  Gain=-1
  Gain2 : Gain  Gain=-1
  Gain3 : Gain  Gain=-1
  "Lge, e 2 gear" : sharedtransform/Rotation Angles to Direction Cosine Matrix  rotationOrder=XYZ  aMode=aMode
  M_fgr scp : Scope
  Math Function : Math  Operator=transpose  SignedPower=on
  Math Function1 : Math  Operator=transpose  SignedPower=on
  Math Function2 : Math  Operator=transpose  SignedPower=on
  Mux{,1..3} (4 alike) : Mux  Inputs=3
  Product{1,4..6} (4 alike) : Product
  Product{2..3,7..11} (7 alike) : Product  Multiplication=Matrix(*)
  Selector1 : Selector  InputPortWidth=3  IndexOptions=Index vector (dialog)  Indices=2  OutputSizes=1
  Selector2 : Selector  InputPortWidth=3  IndexOptions=Index vector (dialog)  Indices=1  OutputSizes=1
  Selector{3..7} (5 alike) : Selector  InputPortWidth=3  IndexOptions=Index vector (dialog)  Indices=3  OutputSizes=1
  Sum{1..3,5,7} (5 alike) : Sum  Inputs=|++
  Sum4 : Sum  Inputs=|+-
  Sum6 : Sum  Inputs=-+|
  Switch1 : Switch  SaturateOnIntegerOverflow=off  InputSameDT=off
  Trigonometric Function : Trigonometry  Operator=atan
  beta fgl{,1..3} (4 alike) : Scope
  hrel_fgl : Scope
  F_fgl : Outport  VectorParamsAs1DForOutWhenUnconnected=off
  M_fgl : Outport  Port=2  VectorParamsAs1DForOutWhenUnconnected=off
  wires:
  Selector5/1 -> Sum2/2
  Constant3/1 -> Mux/1, Mux/2
  Bus Selector/3 -> Sum7/1  "<Vb>"
  Product3/1 -> beta fgl1/1, Selector2/1, Selector1/1, Gain1/1
  Cross Product/1 -> M_fgl/1, M_fgr scp/1
  Math Function2/1 -> Product7/1, Product9/1
  Product5/1 -> Mux1/2
  dg/1 -> Mux2/3, Sum5/1
  Constant7/1 -> Product4/2
  Sum5/1 -> Mux3/3
  Constant5/1 -> Mux2/2, Mux2/1
  Sum1/1 -> Product8/2
  Constant4/1 -> Product5/1
  Selector4/1 -> Sum3/2
  Sum3/1 -> Switch1/3
  Constant11/1 -> Mux3/2, Mux3/1
  Mux/1 -> Sum1/1
  Mux3/1 -> "Lge, e 2 gear"/1
  Switch1/1 -> Gain2/1, F_in_earth scp1/1, Mux/3  "Fz_fgl"
  Constant1/1 -> Mux1/1
  Product6/1 -> Selector4/1
  Product10/1 -> Product7/2
  Selector3/1 -> Sum5/2
  "Lge, e 2 gear"/1 -> Product3/1, Math Function2/1
  Divide/1 -> Trigonometric Function/1
  Cross Product1/1 -> Sum7/2
  Constant6/1 -> Switch1/1
  Sum2/1 -> beta fgl3/1, Product5/2
  Product9/1 -> Sum1/2, F_in_earth scp/1  "F_in_earth"
  Product4/1 -> Sum3/1
  Selector1/1 -> Divide/1
  Product1/1 -> Product9/2, F_in_gear scp/1  "F_in_gear"
  Gain2/1 -> Product1/1
  Selector2/1 -> Divide/2
  Mux1/1 -> Product1/2  "F_in_gear"
  Gain1/1 -> Product6/2
  Constant9/1 -> Mux1/3
  Sum7/1 -> Product2/2
  Product8/1 -> F_fgl/1, F_fgl scp/1, Cross Product/2  "F_support_in_b"
  Mux2/1 -> Product10/2
  Bus Selector/5 -> Selector3/1  "<Euler>"
  Trigonometric Function/1 -> Sum2/1, beta fgl/1  "beta"
  Constant8/1 -> Product6/1
  Math Function1/1 -> Product2/1
  Product2/1 -> beta fgl2/1, Product3/2
  Bus Selector/4 -> Cross Product1/1  "<pqr>"
  Product7/1 -> Selector5/1
  Sum4/1 -> Product4/1, Switch1/2, hrel_fgl/1  "hrel_fgl"
  Bus Selector/1 -> Selector7/1  "<Xe>"
  Constant15/1 -> Sum6/1
  Selector6/1 -> Sum4/2  "z_cg2fgl_in_e_free"
  Product11/1 -> Selector6/1
  Selector7/1 -> Gain3/1
  Bus Selector/2 -> Product10/1, Product8/1, Math Function1/1, Math Function/1  "<DCM_be>"
  Math Function/1 -> Product11/1
  Gain3/1 -> Sum6/2
  Constant2/1 -> Cross Product/1, Product11/2, Cross Product1/2
  Sum6/1 -> Sum4/1  "hrel_cg"
  PlantData/1 -> Bus Selector/1

== system eVTOL_PX4_2023b/Subsystem1/airframe/force moment/Gear&FM in body axis/F&M  Front Gear Right ==
  PlantData : Inport
  dg : Inport  Port=2
  Bus Selector : BusSelector  OutputSignals=Xe,DCM_be,Vb,pqr,Euler
  Constant1 : Constant  Value=General.CD0_gear_taxi
  Constant{3,5..6,9,11} (5 alike) : Constant  Value=0
  Constant15 : Constant  Value=InitData.h_runway
  Constant2 : Constant  Value=General.pos_fgr
  Constant4 : Constant  Value=General.Kb
  Constant7 : Constant  Value=General.Kf
  Constant8 : Constant  Value=General.Cf
  Cross Product : vrlib/Utilities/Cross Product
  Cross Product1 : vrlib/Utilities/Cross Product
  Divide : Product  Inputs=*/
  F_fgl scp : Scope
  F_in_earth scp : Scope
  F_in_earth scp1 : Scope
  F_in_gear scp : Scope
  Gain1 : Gain  Gain=-1
  Gain2 : Gain  Gain=-1
  Gain3 : Gain  Gain=-1
  "Lge, e 2 gear" : sharedtransform/Rotation Angles to Direction Cosine Matrix  rotationOrder=XYZ  aMode=aMode
  M_fgr scp : Scope
  Math Function : Math  Operator=transpose  SignedPower=on
  Math Function1 : Math  Operator=transpose  SignedPower=on
  Math Function2 : Math  Operator=transpose  SignedPower=on
  Mux{,1..3} (4 alike) : Mux  Inputs=3
  Product{1,4..6} (4 alike) : Product
  Product{2..3,7..11} (7 alike) : Product  Multiplication=Matrix(*)
  Selector1 : Selector  InputPortWidth=3  IndexOptions=Index vector (dialog)  Indices=2  OutputSizes=1
  Selector2 : Selector  InputPortWidth=3  IndexOptions=Index vector (dialog)  Indices=1  OutputSizes=1
  Selector{3..7} (5 alike) : Selector  InputPortWidth=3  IndexOptions=Index vector (dialog)  Indices=3  OutputSizes=1
  Sum{1..3,5,7} (5 alike) : Sum  Inputs=|++
  Sum4 : Sum  Inputs=|+-
  Sum6 : Sum  Inputs=-+|
  Switch1 : Switch  SaturateOnIntegerOverflow=off  InputSameDT=off
  Trigonometric Function : Trigonometry  Operator=atan
  beta fgl{,1..3} (4 alike) : Scope
  hrel_fgl : Scope
  F_fgl : Outport  VectorParamsAs1DForOutWhenUnconnected=off
  M_fgl : Outport  Port=2  VectorParamsAs1DForOutWhenUnconnected=off
  wires:
  Selector5/1 -> Sum2/2
  Constant3/1 -> Mux/1, Mux/2
  Bus Selector/3 -> Sum7/1  "<Vb>"
  Product3/1 -> beta fgl1/1, Selector2/1, Selector1/1, Gain1/1
  Cross Product/1 -> M_fgl/1, M_fgr scp/1
  Math Function2/1 -> Product7/1, Product9/1
  Product5/1 -> Mux1/2
  dg/1 -> Mux2/3, Sum5/1
  Constant7/1 -> Product4/2
  Sum5/1 -> Mux3/3
  Constant5/1 -> Mux2/2, Mux2/1
  Sum1/1 -> Product8/2
  Constant4/1 -> Product5/1
  Selector4/1 -> Sum3/2
  Sum3/1 -> Switch1/3
  Constant11/1 -> Mux3/2, Mux3/1
  Mux/1 -> Sum1/1
  Mux3/1 -> "Lge, e 2 gear"/1
  Switch1/1 -> Gain2/1, F_in_earth scp1/1, Mux/3  "Fz_fgl"
  Constant1/1 -> Mux1/1
  Product6/1 -> Selector4/1
  Product10/1 -> Product7/2
  Selector3/1 -> Sum5/2
  "Lge, e 2 gear"/1 -> Product3/1, Math Function2/1
  Divide/1 -> Trigonometric Function/1
  Cross Product1/1 -> Sum7/2
  Constant6/1 -> Switch1/1
  Sum2/1 -> beta fgl3/1, Product5/2
  Product9/1 -> Sum1/2, F_in_earth scp/1  "F_in_earth"
  Product4/1 -> Sum3/1
  Selector1/1 -> Divide/1
  Product1/1 -> Product9/2, F_in_gear scp/1  "F_in_gear"
  Gain2/1 -> Product1/1
  Selector2/1 -> Divide/2
  Mux1/1 -> Product1/2  "F_in_gear"
  Gain1/1 -> Product6/2
  Constant9/1 -> Mux1/3
  Sum7/1 -> Product2/2
  Product8/1 -> F_fgl/1, F_fgl scp/1, Cross Product/2  "F_support_in_b"
  Mux2/1 -> Product10/2
  Bus Selector/5 -> Selector3/1  "<Euler>"
  Trigonometric Function/1 -> Sum2/1, beta fgl/1  "beta"
  Constant8/1 -> Product6/1
  Math Function1/1 -> Product2/1
  Product2/1 -> beta fgl2/1, Product3/2
  Bus Selector/4 -> Cross Product1/1  "<pqr>"
  Product7/1 -> Selector5/1
  Sum4/1 -> Product4/1, Switch1/2, hrel_fgl/1  "hrel_fgl"
  Bus Selector/1 -> Selector7/1  "<Xe>"
  Constant15/1 -> Sum6/1
  Selector6/1 -> Sum4/2  "z_cg2fgl_in_e_free"
  Product11/1 -> Selector6/1
  Selector7/1 -> Gain3/1
  Bus Selector/2 -> Product10/1, Product8/1, Math Function1/1, Math Function/1  "<DCM_be>"
  Math Function/1 -> Product11/1
  Gain3/1 -> Sum6/2
  Constant2/1 -> Cross Product/1, Product11/2, Cross Product1/2
  Sum6/1 -> Sum4/1  "hrel_cg"
  PlantData/1 -> Bus Selector/1

== system eVTOL_PX4_2023b/Subsystem1/airframe/force moment/Gear&FM in body axis/F&M  Main Gear Left ==
  PlantData : Inport
  dg : Inport  Port=2
  Bus Selector : BusSelector  OutputSignals=Xe,DCM_be,Vb,pqr,Euler
  Constant1 : Constant  Value=General.CD0_gear_taxi
  Constant{3,5..6,9,11} (5 alike) : Constant  Value=0
  Constant15 : Constant  Value=InitData.h_runway
  Constant2 : Constant  Value=General.pos_mgl
  Constant4 : Constant  Value=General.Kb
  Constant7 : Constant  Value=General.Kf
  Constant8 : Constant  Value=General.Cf
  Cross Product : vrlib/Utilities/Cross Product
  Cross Product1 : vrlib/Utilities/Cross Product
  Divide : Product  Inputs=*/
  F_fgl scp : Scope
  F_in_earth scp : Scope
  F_in_earth scp1 : Scope
  F_in_gear scp : Scope
  Gain1 : Gain  Gain=-1
  Gain2 : Gain  Gain=-1
  Gain3 : Gain  Gain=-1
  "Lge, e 2 gear" : sharedtransform/Rotation Angles to Direction Cosine Matrix  rotationOrder=XYZ  aMode=aMode
  M_fgr scp : Scope
  Math Function : Math  Operator=transpose  SignedPower=on
  Math Function1 : Math  Operator=transpose  SignedPower=on
  Math Function2 : Math  Operator=transpose  SignedPower=on
  Mux{,1..3} (4 alike) : Mux  Inputs=3
  Product{1,4..6} (4 alike) : Product
  Product{2..3,7..11} (7 alike) : Product  Multiplication=Matrix(*)
  Selector1 : Selector  InputPortWidth=3  IndexOptions=Index vector (dialog)  Indices=2  OutputSizes=1
  Selector2 : Selector  InputPortWidth=3  IndexOptions=Index vector (dialog)  Indices=1  OutputSizes=1
  Selector{3..7} (5 alike) : Selector  InputPortWidth=3  IndexOptions=Index vector (dialog)  Indices=3  OutputSizes=1
  Sum{1..3,5,7} (5 alike) : Sum  Inputs=|++
  Sum4 : Sum  Inputs=|+-
  Sum6 : Sum  Inputs=-+|
  Switch1 : Switch  SaturateOnIntegerOverflow=off  InputSameDT=off
  Trigonometric Function : Trigonometry  Operator=atan
  beta fgl{,1..3} (4 alike) : Scope
  hrel_fgl : Scope
  F_fgl : Outport  VectorParamsAs1DForOutWhenUnconnected=off
  M_fgl : Outport  Port=2  VectorParamsAs1DForOutWhenUnconnected=off
  wires:
  Selector5/1 -> Sum2/2
  Constant3/1 -> Mux/1, Mux/2
  Bus Selector/3 -> Sum7/1  "<Vb>"
  Product3/1 -> beta fgl1/1, Selector2/1, Selector1/1, Gain1/1
  Cross Product/1 -> M_fgl/1, M_fgr scp/1
  Math Function2/1 -> Product7/1, Product9/1
  Product5/1 -> Mux1/2
  dg/1 -> Mux2/3, Sum5/1
  Constant7/1 -> Product4/2
  Sum5/1 -> Mux3/3
  Constant5/1 -> Mux2/2, Mux2/1
  Sum1/1 -> Product8/2
  Constant4/1 -> Product5/1
  Selector4/1 -> Sum3/2
  Sum3/1 -> Switch1/3
  Constant11/1 -> Mux3/2, Mux3/1
  Mux/1 -> Sum1/1
  Mux3/1 -> "Lge, e 2 gear"/1
  Switch1/1 -> Gain2/1, F_in_earth scp1/1, Mux/3  "Fz_fgl"
  Constant1/1 -> Mux1/1
  Product6/1 -> Selector4/1
  Product10/1 -> Product7/2
  Selector3/1 -> Sum5/2
  "Lge, e 2 gear"/1 -> Product3/1, Math Function2/1
  Divide/1 -> Trigonometric Function/1
  Cross Product1/1 -> Sum7/2
  Constant6/1 -> Switch1/1
  Sum2/1 -> beta fgl3/1, Product5/2
  Product9/1 -> Sum1/2, F_in_earth scp/1  "F_in_earth"
  Product4/1 -> Sum3/1
  Selector1/1 -> Divide/1
  Product1/1 -> Product9/2, F_in_gear scp/1  "F_in_gear"
  Gain2/1 -> Product1/1
  Selector2/1 -> Divide/2
  Mux1/1 -> Product1/2  "F_in_gear"
  Gain1/1 -> Product6/2
  Constant9/1 -> Mux1/3
  Sum7/1 -> Product2/2
  Product8/1 -> F_fgl/1, F_fgl scp/1, Cross Product/2  "F_support_in_b"
  Mux2/1 -> Product10/2
  Bus Selector/5 -> Selector3/1  "<Euler>"
  Trigonometric Function/1 -> Sum2/1, beta fgl/1  "beta"
  Constant8/1 -> Product6/1
  Math Function1/1 -> Product2/1
  Product2/1 -> beta fgl2/1, Product3/2
  Bus Selector/4 -> Cross Product1/1  "<pqr>"
  Product7/1 -> Selector5/1
  Sum4/1 -> Product4/1, Switch1/2, hrel_fgl/1  "hrel_fgl"
  Bus Selector/1 -> Selector7/1  "<Xe>"
  Constant15/1 -> Sum6/1
  Selector6/1 -> Sum4/2  "z_cg2fgl_in_e_free"
  Product11/1 -> Selector6/1
  Selector7/1 -> Gain3/1
  Bus Selector/2 -> Product10/1, Product8/1, Math Function1/1, Math Function/1  "<DCM_be>"
  Math Function/1 -> Product11/1
  Gain3/1 -> Sum6/2
  Constant2/1 -> Cross Product/1, Product11/2, Cross Product1/2
  Sum6/1 -> Sum4/1  "hrel_cg"
  PlantData/1 -> Bus Selector/1
